simulink model "experiment_1_lab_05_c"  (Simulink 7.1)
settings: Solver=ode45  StartTime=0.0  StopTime=10.0  RelTol=1e-3
InitFcn:
  | R1=2;
  | R2=4;
  | L1=0.5;
  | L2=1;
  | C=3/8;
  | A=[-R1/L1,0,-1/L1;0,-R2/L2,1/L2;1/C,-1/C,0];
  | B= [1/L1;0;0];
  | C=[0,R2,0;1,0,0;0,1,0;0,0,1];
  | D=[0;0;0;0];
  | Q=[0,4,0;0,-16,4;(32/3),(160/3),-16];
  | AB=Q*A*inv(Q);
  | BB=Q*B;
  | CB=C*inv(Q);
  | DB=[0;0;0;0];
settings Model: Creator=ALUNO  LastModifiedBy=ALUNO

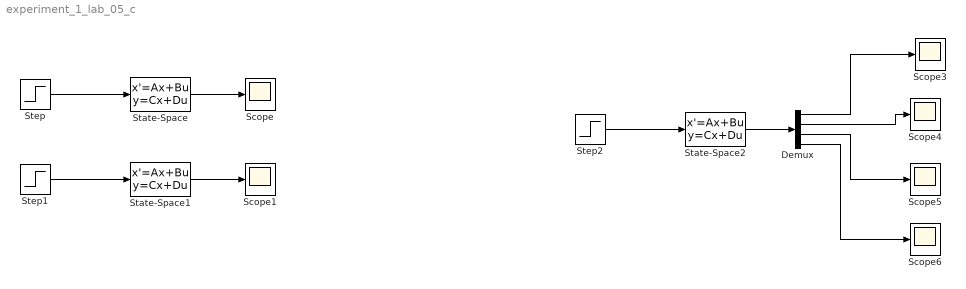
== system experiment_1_lab_05_c ==
  Demux : Demux
  Scope{,1,3..6} (6 alike) : Scope
      Scope3 settings: SaveName=ScopeData4
      Scope4 settings: SaveName=ScopeData5
      Scope5 settings: SaveName=ScopeData6
      Scope6 settings: SaveName=ScopeData3
  State-Space : StateSpace  A=AB  B=BB  C=CB  D=DB
  State-Space1 : StateSpace  A=A  B=B  C=C  D=D
  State-Space2 : StateSpace  A=AB  B=BB  C=CB  D=DB
  Step : Step  Time=0  SampleTime=0
  Step1 : Step  Time=0  SampleTime=0
  Step2 : Step  Time=0  SampleTime=0
  wires:
  Step/1 -> State-Space/1
  State-Space/1 -> Scope/1
  Step1/1 -> State-Space1/1
  State-Space1/1 -> Scope1/1
  Step2/1 -> State-Space2/1
  State-Space2/1 -> Demux/1
  Demux/1 -> Scope3/1
  Demux/2 -> Scope4/1
  Demux/3 -> Scope5/1
  Demux/4 -> Scope6/1
